simulink model "Simulink_Vortex"  (R2015b)
settings: Solver=ode3  StartTime=0.0  StopTime=20.603  FixedStep=0.016666  RelTol=1e-3
InitFcn:
  | state=0
values from neighbouring files (symbols this model uses):
  acc = 2    [sim_ExoTeR_VORTEX.m]
  mode = 0    [sim_ExoTeR_VORTEX.m]
libraries: simulink x6, Vortex x1
settings Model: Creator=pablorm  LastModifiedBy=gonzalopd96
settings RTWCC: PostCodeGenCommand=PrepareVortexForSimulinkCoder(buildInfo)

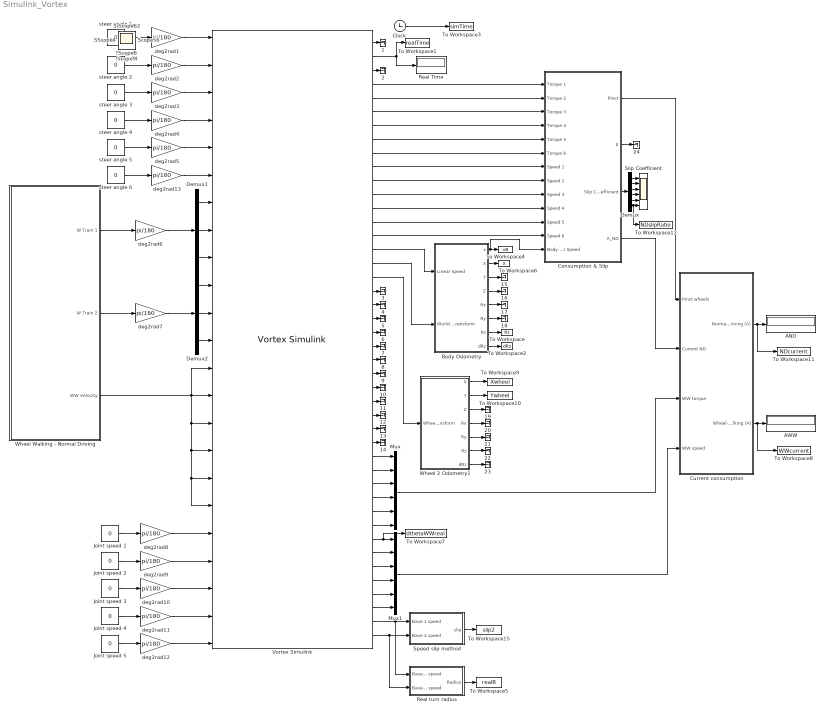
== system Simulink_Vortex ==
  {1..24} (24 alike) : Terminator
  AND : Display
  AWW : Display
  Body Odometry : Subsystem
  Clock : Clock
  Consumption & Slip : Subsystem
  Current consumption : Subsystem
  Demux : Demux  Outputs=6
  Demux1 : Demux  Outputs=3
  Demux2 : Demux  Outputs=3
  Joint speed {1..5} (5 alike) : Constant  Value=0
  Mux : Mux  Inputs=6
  Mux1 : Mux  Inputs=6
  Real Time : Display
  "Real turn radius " : Subsystem
  Slip Coefficient : Scope  NumInputPorts=6
  Speed slip method : Subsystem
  To Workspace : ToWorkspace  VariableName=Rz  SampleTime=-1
  To Workspace1 : ToWorkspace  VariableName=realTime  SampleTime=-1
  To Workspace10 : ToWorkspace  VariableName=Ywheel  SampleTime=-1
  To Workspace11 : ToWorkspace  VariableName=NDcurrent  SampleTime=-1
  To Workspace12 : ToWorkspace  VariableName=NDslipRatio  SampleTime=-1
  To Workspace15 : ToWorkspace  VariableName=slip2  SampleTime=-1
  To Workspace2 : ToWorkspace  VariableName=dRz  SampleTime=-1
  To Workspace3 : ToWorkspace  VariableName=simTime  SampleTime=-1
  To Workspace4 : ToWorkspace  VariableName=vB  SampleTime=-1
  To Workspace5 : ToWorkspace  VariableName=realR  SampleTime=-1
  To Workspace6 : ToWorkspace  VariableName=X  SampleTime=-1
  To Workspace7 : ToWorkspace  VariableName=dthetaWWreal  SampleTime=-1
      settings: Save2DSignal=2-D array (concatenate along first dimension)
  To Workspace8 : ToWorkspace  VariableName=WWcurrent  SampleTime=-1
  To Workspace9 : ToWorkspace  VariableName=Xwheel  SampleTime=-1
  Vortex Simulink : Vortex/Vortex Simulink  ip='127.0.0.1'  port='736'  path='C:\Users\gonzalopd96\Documents\VortexSimulink\Simulink\Simulink configurations\Rover_config.json'  display=image(imread('logo.jpg'), [0, 0, 48, 48]);fprintf('\n\n\nMy Model');port_label('input',1,'Steer1Angle');port_label('input',2,'Steer2Angle');port_label('input',3,'Steer3Angle');port_label('input',4,'Steer4Angle');port_label('input',5,'Steer5Angle');port_label('input',6,'Steer6Angle');port_label('input',7,'Speed1');port_label('input',8,'Speed2');port_label('input',9,'Speed3');port_label('input',10,'Speed4');port_label('input',11,'Speed5');port_label('input',12,'Speed6');port_label('input',13,'WJ1');port_label('input',14,'WJ2');port_label('input',15,'WJ3');port_label('input',16,'WJ4');port_label('input',17,'WJ5');port_label('input',18,'WJ6');port_label('input',19,'Joint speed 1');port_label('input',20,'Joint speed 2');port_label('input',21,'Joint speed 3');port_label('input',22,'Joint speed 4');port_label('input',23,'Joint speed 5');port_label('output',1,'Status');port_label('output',2,'Time');port_label('output',3,'FrameIndex');port_label('output',4,'Torque1');port_label('output',5,'Torque2');port_label('output',6,'Torque3');port_label('output',7,'Torque4');port_label('output',8,'Torque5');port_label('output',9,'Torque6');port_label('output',10,'Speed1');port_label('output',11,'Speed2');port_label('output',12,'Speed3');port_label('output',13,'Speed4');port_label('output',14,'Speed5');port_label('output',15,'Speed6');port_label('output',16,'Lineal Speed');port_label('output',17,'World Transform');port_label('output',18,'Wheel Transform');port_label('output',19,'Motor Transform');port_label('output',20,'PosJ1');port_label('output',21,'PosJ2');port_label('output',22,'PosJ3');port_label('output',23,'PosJ4');port_label('output',24,'PosJ5');port_label('output',25,'Steer1');port_label('output',26,'Steer2');port_label('output',27,'Steer3');port_label('output',28,'Steer4');port_label('output',29,'Steer5');port_label('output',30,'Steer6');port_label('output',31,'WW Torque 1');port_label('output',32,'WW Torque 2');port_label('output',33,'WW Torque 3');port_label('output',34,'WW Torque 4');port_label('output',35,'WW Torque 5');port_label('output',36,'WW Torque 6');port_label('output',37,'WW Speed 1');port_label('output',38,'WW Speed 2');port_label('output',39,'WW Speed 3');port_label('output',40,'WW Speed 4');port_label('output',41,'WW Speed 5');port_label('output',42,'WW Speed 6');port_label('output',43,'RS position');port_label('output',44,'LS position');  SynchronizationMechanism=Active wait at each step  WaitVortex=on
  Wheel 2 Odometry1 : Subsystem
  Wheel Walking - Normal Driving : Subsystem
  deg2rad{1..13} (13 alike) : Gain  Gain=pi/180
  steer angle {1..6} (6 alike) : Constant  Value=0
  Scope{,1..6,8..17} (17 alike) : Scope
  wires:
  deg2rad4/1 -> Vortex Simulink/4
  deg2rad3/1 -> Vortex Simulink/3
  deg2rad2/1 -> Vortex Simulink/2
  deg2rad5/1 -> Vortex Simulink/5
  deg2rad13/1 -> Vortex Simulink/6
  Joint speed 1/1 -> deg2rad8/1
  Joint speed 2/1 -> deg2rad9/1
  Joint speed 3/1 -> deg2rad10/1
  Joint speed 4/1 -> deg2rad11/1
  Joint speed 5/1 -> deg2rad12/1
  Vortex Simulink/4 -> Consumption & Slip/1(Torque 1)
  Vortex Simulink/6 -> Consumption & Slip/3(Torque 3)
  Vortex Simulink/7 -> Consumption & Slip/4(Torque 4)
  Vortex Simulink/8 -> Consumption & Slip/5(Torque 5)
  Vortex Simulink/9 -> Consumption & Slip/6(Torque 6)
  Vortex Simulink/10 -> Consumption & Slip/7(Speed 1)
  Vortex Simulink/11 -> Consumption & Slip/8(Speed 2)
  Vortex Simulink/12 -> Consumption & Slip/9(Speed 3)
  Vortex Simulink/13 -> Consumption & Slip/10(Speed 4)
  Vortex Simulink/14 -> Consumption & Slip/11(Speed 5)
  Vortex Simulink/15 -> Consumption & Slip/12(Speed 6)
  Body Odometry/1(v) -> Consumption & Slip/13(Body Linear Speed), To Workspace4/1
  Vortex Simulink/16 -> Body Odometry/1(Linear Speed)
  steer angle 6/1 -> deg2rad13/1
  steer angle 2/1 -> deg2rad2/1
  steer angle 3/1 -> deg2rad3/1
  steer angle 4/1 -> deg2rad4/1
  steer angle 5/1 -> deg2rad5/1
  Wheel Walking - Normal Driving/1(W Train 1) -> deg2rad6/1
  Wheel Walking - Normal Driving/2(W Train 2) -> deg2rad7/1
  Vortex Simulink/17 -> Body Odometry/2(World transform)
  Demux1/3 -> Vortex Simulink/9
  Demux1/2 -> Vortex Simulink/8
  deg2rad6/1 -> Demux1/1
  Demux2/2 -> Vortex Simulink/11
  Demux2/1 -> Vortex Simulink/10
  Demux2/3 -> Vortex Simulink/12
  deg2rad7/1 -> Demux2/1
  Consumption & Slip/3(Slip Coefficient) -> Demux/1
  Demux/1 -> Slip Coefficient/1
  Demux/2 -> Slip Coefficient/2
  Demux/3 -> Slip Coefficient/3
  Demux/4 -> Slip Coefficient/4
  Demux/5 -> Slip Coefficient/5
  Demux/6 -> To Workspace12/1, Slip Coefficient/6
  Vortex Simulink/2 -> To Workspace1/1, Real Time/1
  Demux1/1 -> Vortex Simulink/7
  Vortex Simulink/5 -> Consumption & Slip/2(Torque 2)
  Clock/1 -> To Workspace3/1
  Body Odometry/2(X) -> To Workspace6/1
  Body Odometry/7(Rz) -> To Workspace/1
  Body Odometry/8(dRz) -> To Workspace2/1
  Wheel 2 Odometry1/2(Y) -> To Workspace10/1
  Wheel 2 Odometry1/1(X) -> To Workspace9/1
  Speed slip method/1(slip) -> To Workspace15/1
  Consumption & Slip/1(PInst) -> Current consumption/1(Pinst wheels)
  Consumption & Slip/4(A_ND) -> Current consumption/2(Current ND)
  Mux/1 -> Current consumption/3(WW torque)
  Mux1/1 -> Current consumption/4(WW speed)
  Current consumption/1(Normal driving (A)) -> To Workspace11/1, AND/1
  Current consumption/2(Wheel-walking (A)) -> To Workspace8/1, AWW/1
  deg2rad1/1 -> Vortex Simulink/1
  steer angle 1/1 -> deg2rad1/1
  Body Odometry/4(Z) -> 16/1
  Body Odometry/6(Ry) -> 18/1
  Body Odometry/5(Rx) -> 17/1
  Body Odometry/3(Y) -> 15/1
  Consumption & Slip/2(P) -> 24/1
  Vortex Simulink/1 -> 1/1
  Vortex Simulink/3 -> 2/1
  Wheel 2 Odometry1/3(Z) -> 19/1
  Wheel 2 Odometry1/4(Rx) -> 20/1
  Wheel 2 Odometry1/5(Ry) -> 21/1
  Wheel 2 Odometry1/6(Rz) -> 22/1
  Wheel 2 Odometry1/7(dRz) -> 23/1
  "Real turn radius "/1(Radius) -> To Workspace5/1
  Wheel Walking - Normal Driving/3(WW Velocity) -> Vortex Simulink/14, Vortex Simulink/13, Vortex Simulink/15, Vortex Simulink/16, Vortex Simulink/18, Vortex Simulink/17
  deg2rad8/1 -> Vortex Simulink/19
  deg2rad9/1 -> Vortex Simulink/20
  deg2rad10/1 -> Vortex Simulink/21
  deg2rad11/1 -> Vortex Simulink/22
  deg2rad12/1 -> Vortex Simulink/23
  Vortex Simulink/43 -> "Real turn radius "/1(Base 1 speed), Speed slip method/1(Base 1 speed)
  Vortex Simulink/44 -> "Real turn radius "/2(Base 2 speed), Speed slip method/2(Base 2 speed)
  Vortex Simulink/18 -> Wheel 2 Odometry1/1(Wheel transform)
  Vortex Simulink/19 -> 3/1
  Vortex Simulink/20 -> 4/1
  Vortex Simulink/21 -> 5/1
  Vortex Simulink/22 -> 6/1
  Vortex Simulink/23 -> 7/1
  Vortex Simulink/24 -> 8/1
  Vortex Simulink/25 -> 9/1
  Vortex Simulink/26 -> 10/1
  Vortex Simulink/27 -> 11/1
  Vortex Simulink/28 -> 12/1
  Vortex Simulink/29 -> 13/1
  Vortex Simulink/30 -> 14/1
  Vortex Simulink/36 -> Mux/6
  Vortex Simulink/35 -> Mux/5
  Vortex Simulink/34 -> Mux/4
  Vortex Simulink/33 -> Mux/3
  Vortex Simulink/32 -> Mux/2
  Vortex Simulink/31 -> Mux/1
  Vortex Simulink/38 -> Mux1/2
  Vortex Simulink/39 -> Mux1/3
  Vortex Simulink/40 -> Mux1/4
  Vortex Simulink/41 -> Mux1/5
  Vortex Simulink/42 -> Mux1/6
  Vortex Simulink/37 -> To Workspace7/1, Mux1/1

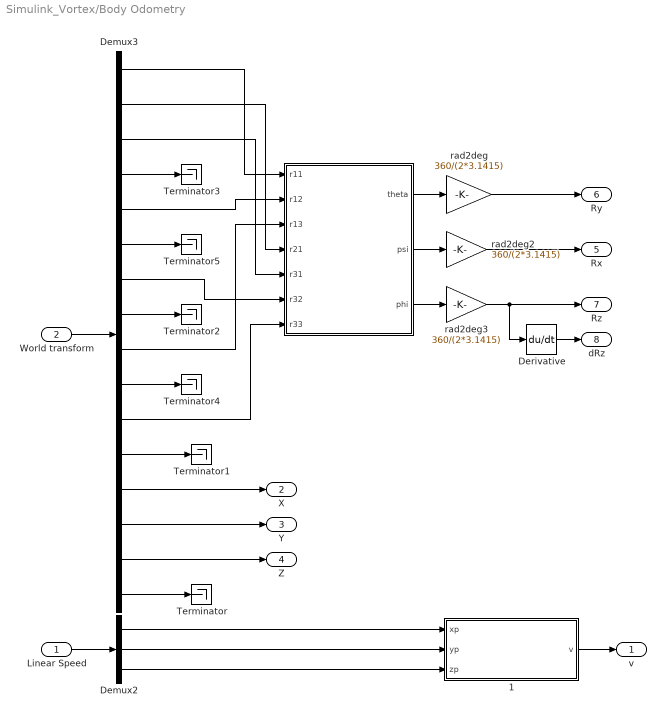
== system Simulink_Vortex/Body Odometry ==
  Linear Speed : Inport
  World transform : Inport  Port=2
  " " : MATLAB Function  TreatAsAtomicUnit=on
  1 : MATLAB Function  TreatAsAtomicUnit=on
  Demux2 : Demux  Outputs=3
  Demux3 : Demux  Outputs=16
  Derivative : Derivative
  Terminator{,1..5} (6 alike) : Terminator
  rad2deg : Gain  Gain=360/(2*3.1415)
  rad2deg2 : Gain  Gain=360/(2*3.1415)
  rad2deg3 : Gain  Gain=360/(2*3.1415)
  v : Outport
  X : Outport  Port=2
  Y : Outport  Port=3
  Z : Outport  Port=4
  Rx : Outport  Port=5
  Ry : Outport  Port=6
  Rz : Outport  Port=7
  dRz : Outport  Port=8
  wires:
  World transform/1 -> Demux3/1
  Demux3/13 -> X/1
  Demux3/14 -> Y/1
  Demux3/15 -> Z/1
  Demux3/7 -> " "/6(r32)
  Demux3/6 -> Terminator5/1
  " "/2(psi) -> rad2deg2/1
  " "/1(theta) -> rad2deg/1
  Demux3/4 -> Terminator3/1
  " "/3(phi) -> rad2deg3/1
  Demux3/12 -> Terminator1/1
  Demux3/16 -> Terminator/1
  rad2deg3/1 -> Derivative/1, Rz/1
  rad2deg2/1 -> Rx/1
  rad2deg/1 -> Ry/1
  Linear Speed/1 -> Demux2/1
  Demux2/1 -> 1/1(xp)
  1/1(v) -> v/1
  Demux2/2 -> 1/2(yp)
  Demux2/3 -> 1/3(zp)
  Derivative/1 -> dRz/1
  Demux3/1 -> " "/1(r11)
  Demux3/2 -> " "/4(r21)
  Demux3/3 -> " "/5(r31)
  Demux3/5 -> " "/2(r12)
  Demux3/8 -> Terminator2/1
  Demux3/9 -> " "/3(r13)
  Demux3/10 -> Terminator4/1
  Demux3/11 -> " "/7(r33)

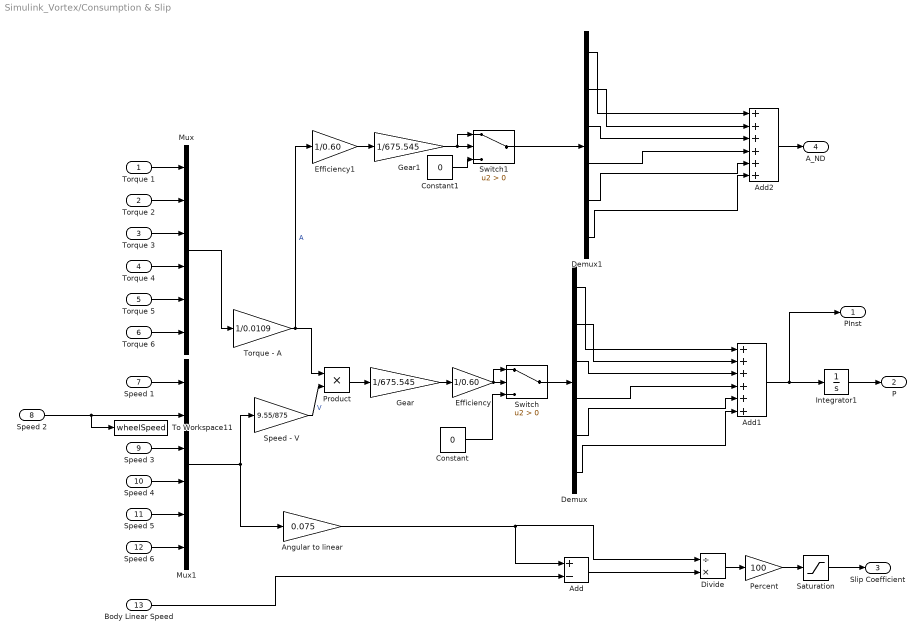
== system Simulink_Vortex/Consumption & Slip ==
  Torque 1 : Inport
  Torque 2 : Inport  Port=2
  Torque 3 : Inport  Port=3
  Torque 4 : Inport  Port=4
  Torque 5 : Inport  Port=5
  Torque 6 : Inport  Port=6
  Speed 1 : Inport  Port=7
  Speed 2 : Inport  Port=8
  Speed 3 : Inport  Port=9
  Speed 4 : Inport  Port=10
  Speed 5 : Inport  Port=11
  Speed 6 : Inport  Port=12
  Body Linear Speed : Inport  Port=13
  Add : Sum  Inputs=+-
  Add1 : Sum  Inputs=++++++
  Add2 : Sum  Inputs=++++++
  Angular to linear : Gain  Gain=0.075
  Constant : Constant  Value=0
  Constant1 : Constant  Value=0
  Demux : Demux  Outputs=6
  Demux1 : Demux  Outputs=6
  Divide : Product  Inputs=/*
  Efficiency : Gain  Gain=1/0.60
  Efficiency1 : Gain  Gain=1/0.60
  Gear : Gain  Gain=1/675.545
  Gear1 : Gain  Gain=1/675.545
  Integrator1 : Integrator
  Mux : Mux  Inputs=6
  Mux1 : Mux  Inputs=6
  Percent : Gain  Gain=100
  Product : Product
  Saturation : Saturate  UpperLimit=100  LowerLimit=0
  Speed - V : Gain  Gain=9.55/875
  Switch : Switch  Criteria=u2 > Threshold
  Switch1 : Switch  Criteria=u2 > Threshold
  To Workspace11 : ToWorkspace  VariableName=wheelSpeed  SampleTime=-1
  Torque - A : Gain  Gain=1/0.0109
  PInst : Outport
  P : Outport  Port=2
  Slip Coefficient : Outport  Port=3
  A_ND : Outport  Port=4
  wires:
  Torque 4/1 -> Mux/4
  Speed 4/1 -> Mux1/4
  Torque 3/1 -> Mux/3
  Torque 2/1 -> Mux/2
  Speed 6/1 -> Mux1/6
  Efficiency/1 -> Switch/1, Switch/2
  Torque 5/1 -> Mux/5
  Integrator1/1 -> P/1
  Torque 6/1 -> Mux/6
  Torque 1/1 -> Mux/1
  Demux/2 -> Add1/2
  Add1/1 -> PInst/1, Integrator1/1
  Torque - A/1 -> Product/1, Efficiency1/1  "A"
  Speed 1/1 -> Mux1/1
  Demux/4 -> Add1/4
  Speed 5/1 -> Mux1/5
  Demux/6 -> Add1/6
  Demux/3 -> Add1/3
  Speed - V/1 -> Product/2  "V"
  Speed 3/1 -> Mux1/3
  Demux/5 -> Add1/5
  Demux/1 -> Add1/1
  Mux1/1 -> Angular to linear/1, Speed - V/1
  Body Linear Speed/1 -> Add/2
  Divide/1 -> Percent/1
  Percent/1 -> Saturation/1
  Saturation/1 -> Slip Coefficient/1
  Add/1 -> Divide/2
  Angular to linear/1 -> Add/1, Divide/1
  Mux/1 -> Torque - A/1
  Switch/1 -> Demux/1
  Constant/1 -> Switch/3
  Product/1 -> Gear/1
  Gear/1 -> Efficiency/1
  Demux1/2 -> Add2/2
  Demux1/4 -> Add2/4
  Demux1/6 -> Add2/6
  Demux1/3 -> Add2/3
  Demux1/5 -> Add2/5
  Demux1/1 -> Add2/1
  Add2/1 -> A_ND/1
  Switch1/1 -> Demux1/1
  Constant1/1 -> Switch1/3
  Gear1/1 -> Switch1/1, Switch1/2
  Efficiency1/1 -> Gear1/1
  Speed 2/1 -> To Workspace11/1, Mux1/2

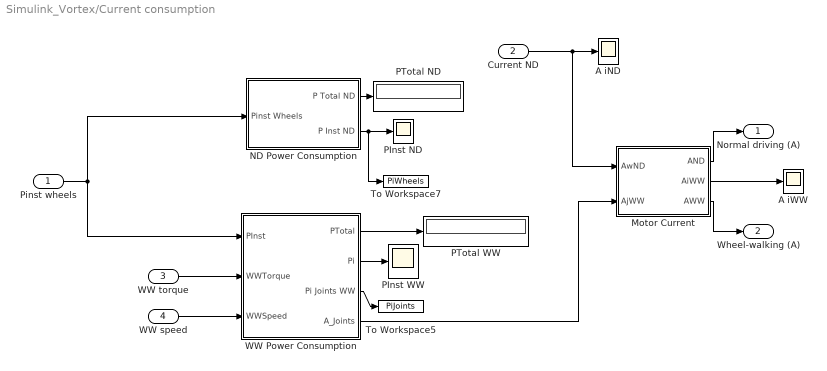
== system Simulink_Vortex/Current consumption ==
  Pinst wheels : Inport
  Current ND : Inport  Port=2
  WW torque : Inport  Port=3
  WW speed : Inport  Port=4
  A iND : Scope
  A iWW : Scope
  Motor Current : Subsystem
  ND Power Consumption : Subsystem
  PInst ND : Scope
  PInst WW : Scope
  PTotal ND : Display
  PTotal WW : Display
  To Workspace5 : ToWorkspace  VariableName=PiJoints  SampleTime=-1
  To Workspace7 : ToWorkspace  VariableName=PiWheels  SampleTime=-1
  WW Power Consumption : Subsystem
  Normal driving (A) : Outport
  Wheel-walking (A) : Outport  Port=2
  wires:
  Pinst wheels/1 -> ND Power Consumption/1(Pinst Wheels), WW Power Consumption/1(PInst)
  WW torque/1 -> WW Power Consumption/2(WWTorque)
  WW Power Consumption/2(Pi) -> PInst WW/1
  WW Power Consumption/1(PTotal) -> PTotal WW/1
  ND Power Consumption/1(P Total ND) -> PTotal ND/1
  ND Power Consumption/2(P Inst ND) -> To Workspace7/1, PInst ND/1
  WW Power Consumption/3(Pi Joints WW) -> To Workspace5/1
  WW speed/1 -> WW Power Consumption/3(WWSpeed)
  Current ND/1 -> Motor Current/1(AwND), A iND/1
  WW Power Consumption/4(A_Joints) -> Motor Current/2(AjWW)
  Motor Current/1(AND) -> Normal driving (A)/1
  Motor Current/3(AWW) -> Wheel-walking (A)/1
  Motor Current/2(AiWW) -> A iWW/1

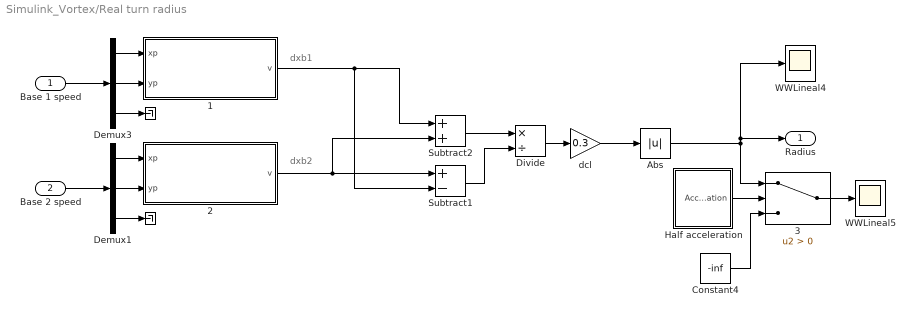
== system Simulink_Vortex/Real turn radius  ==
  note: dxb2
  note: dxb1
  Base 1 speed : Inport
  Base 2 speed : Inport  Port=2
  " " : Terminator
  " " : Terminator
  "     3" : Switch  Criteria=u2 > Threshold
  1 : MATLAB Function  TreatAsAtomicUnit=on
  2 : MATLAB Function  TreatAsAtomicUnit=on
  Abs : Abs
  Constant4 : Constant  Value=-inf
  Demux1 : Demux  Outputs=3
  Demux3 : Demux  Outputs=3
  Divide : Product  Inputs=*/
  Half acceleration : Subsystem
  Subtract1 : Sum  Inputs=+-
  Subtract2 : Sum
  WWLineal4 : Scope
  WWLineal5 : Scope
  dcl : Gain  Gain=0.3
  Radius : Outport
  wires:
  Half acceleration/1(Acceleration) -> "     3"/2
  Divide/1 -> dcl/1
  Constant4/1 -> "     3"/3
  "     3"/1 -> WWLineal5/1
  1/1(v) -> Subtract2/1, Subtract1/2
  dcl/1 -> Abs/1
  Abs/1 -> WWLineal4/1, Radius/1, "     3"/1
  Subtract1/1 -> Divide/2
  Subtract2/1 -> Divide/1
  Base 1 speed/1 -> Demux3/1
  Demux3/2 -> 1/2(yp)
  Demux3/1 -> 1/1(xp)
  Demux3/3 -> " "/1
  Base 2 speed/1 -> Demux1/1
  Demux1/2 -> 2/2(yp)
  Demux1/1 -> 2/1(xp)
  Demux1/3 -> " "/1
  2/1(v) -> Subtract1/1, Subtract2/2

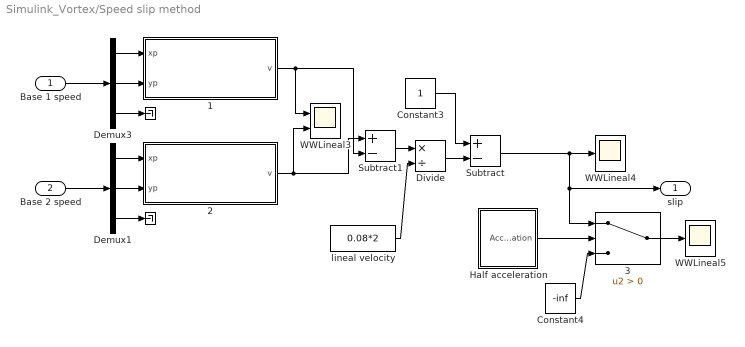
== system Simulink_Vortex/Speed slip method ==
  Base 1 speed : Inport
  Base 2 speed : Inport  Port=2
  " " : Terminator
  " " : Terminator
  "     3" : Switch  Criteria=u2 > Threshold
  1 : MATLAB Function  TreatAsAtomicUnit=on
  2 : MATLAB Function  TreatAsAtomicUnit=on
  Constant3 : Constant
  Constant4 : Constant  Value=-inf
  Demux1 : Demux  Outputs=3
  Demux3 : Demux  Outputs=3
  Divide : Product  Inputs=*/
  Half acceleration : Subsystem
  Subtract : Sum  Inputs=+-
  Subtract1 : Sum  Inputs=+-
  WWLineal3 : Scope  NumInputPorts=2
  WWLineal4 : Scope
  WWLineal5 : Scope
  lineal velocity : Constant  Value=0.08*2
  slip : Outport
  wires:
  Half acceleration/1(Acceleration) -> "     3"/2
  Constant3/1 -> Subtract/1
  Subtract1/1 -> Divide/1
  Divide/1 -> Subtract/2
  lineal velocity/1 -> Divide/2
  Constant4/1 -> "     3"/3
  "     3"/1 -> WWLineal5/1
  2/1(v) -> Subtract1/1, WWLineal3/2
  Subtract/1 -> WWLineal4/1, slip/1, "     3"/1
  1/1(v) -> Subtract1/2, WWLineal3/1
  Base 1 speed/1 -> Demux3/1
  Demux3/2 -> 1/2(yp)
  Demux3/1 -> 1/1(xp)
  Demux3/3 -> " "/1
  Base 2 speed/1 -> Demux1/1
  Demux1/2 -> 2/2(yp)
  Demux1/1 -> 2/1(xp)
  Demux1/3 -> " "/1

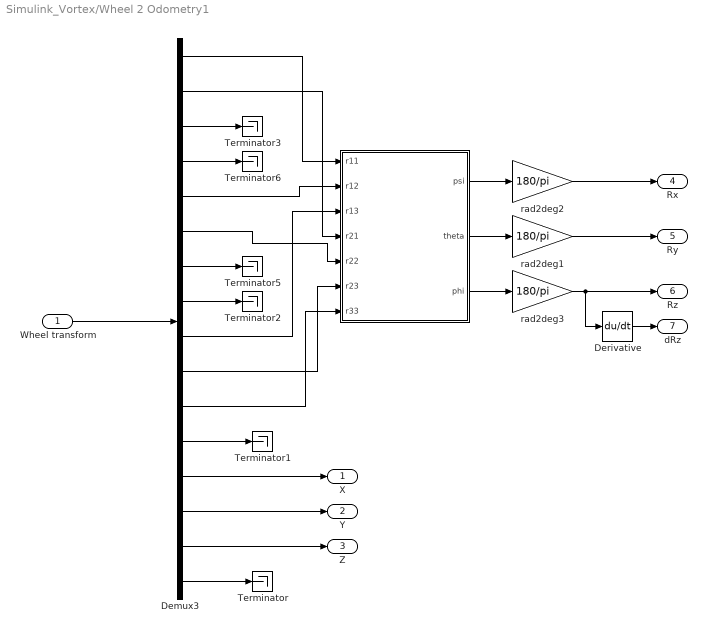
== system Simulink_Vortex/Wheel 2 Odometry1 ==
  Wheel transform : Inport
  " " : MATLAB Function  TreatAsAtomicUnit=on
  Demux3 : Demux  Outputs=16
  Derivative : Derivative
  Terminator{,1..3,5..6} (6 alike) : Terminator
  rad2deg1 : Gain  Gain=180/pi
  rad2deg2 : Gain  Gain=180/pi
  rad2deg3 : Gain  Gain=180/pi
  X : Outport
  Y : Outport  Port=2
  Z : Outport  Port=3
  Rx : Outport  Port=4
  Ry : Outport  Port=5
  Rz : Outport  Port=6
  dRz : Outport  Port=7
  wires:
  Derivative/1 -> dRz/1
  rad2deg1/1 -> Ry/1
  rad2deg2/1 -> Rx/1
  rad2deg3/1 -> Rz/1, Derivative/1
  Demux3/16 -> Terminator/1
  " "/3(phi) -> rad2deg3/1
  " "/2(theta) -> rad2deg1/1
  " "/1(psi) -> rad2deg2/1
  Demux3/15 -> Z/1
  Demux3/14 -> Y/1
  Demux3/13 -> X/1
  Wheel transform/1 -> Demux3/1
  Demux3/12 -> Terminator1/1
  Demux3/8 -> Terminator2/1
  Demux3/1 -> " "/1(r11)
  Demux3/2 -> " "/4(r21)
  Demux3/3 -> Terminator3/1
  Demux3/4 -> Terminator6/1
  Demux3/5 -> " "/2(r12)
  Demux3/6 -> " "/5(r22)
  Demux3/7 -> Terminator5/1
  Demux3/9 -> " "/3(r13)
  Demux3/10 -> " "/6(r23)
  Demux3/11 -> " "/7(r33)

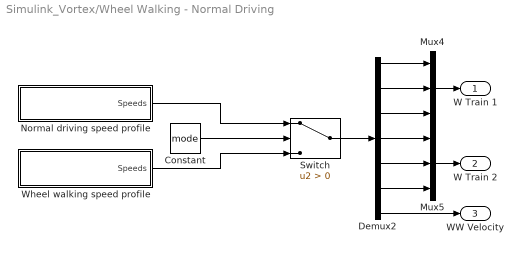
== system Simulink_Vortex/Wheel Walking - Normal Driving ==
  Constant : Constant  Value=mode
  Demux2 : Demux  Outputs=7
  Mux4 : Mux  Inputs=3
  Mux5 : Mux  Inputs=3
  Normal driving speed profile : Subsystem
  Switch : Switch  Criteria=u2 > Threshold
  Wheel walking speed profile : Subsystem
  W Train 1 : Outport
  W Train 2 : Outport  Port=2
  WW Velocity : Outport  Port=3
  wires:
  Demux2/1 -> Mux4/1
  Demux2/2 -> Mux4/2
  Demux2/3 -> Mux4/3
  Demux2/6 -> Mux5/3
  Demux2/5 -> Mux5/2
  Demux2/4 -> Mux5/1
  Mux4/1 -> W Train 1/1
  Mux5/1 -> W Train 2/1
  Demux2/7 -> WW Velocity/1
  Switch/1 -> Demux2/1
  Normal driving speed profile/1(Speeds) -> Switch/1
  Wheel walking speed profile/1(Speeds) -> Switch/3
  Constant/1 -> Switch/2

== system Simulink_Vortex/Current consumption/Motor Current ==
  AwND : Inport
  AjWW : Inport  Port=2
  Add3 : Sum
  Integrator : Integrator
  Integrator1 : Integrator
  AND : Outport
  AiWW : Outport  Port=2
  AWW : Outport  Port=3
  wires:
  Integrator1/1 -> AWW/1
  AjWW/1 -> Add3/2
  Integrator/1 -> AND/1
  Add3/1 -> AiWW/1, Integrator1/1
  AwND/1 -> Integrator/1, Add3/1

== system Simulink_Vortex/Current consumption/ND Power Consumption ==
  Pinst Wheels : Inport
  Gain : Gain
  Integrator : Integrator
  P Total ND : Outport
  P Inst ND : Outport  Port=2
  wires:
  Pinst Wheels/1 -> P Inst ND/1, Gain/1
  Gain/1 -> Integrator/1
  Integrator/1 -> P Total ND/1

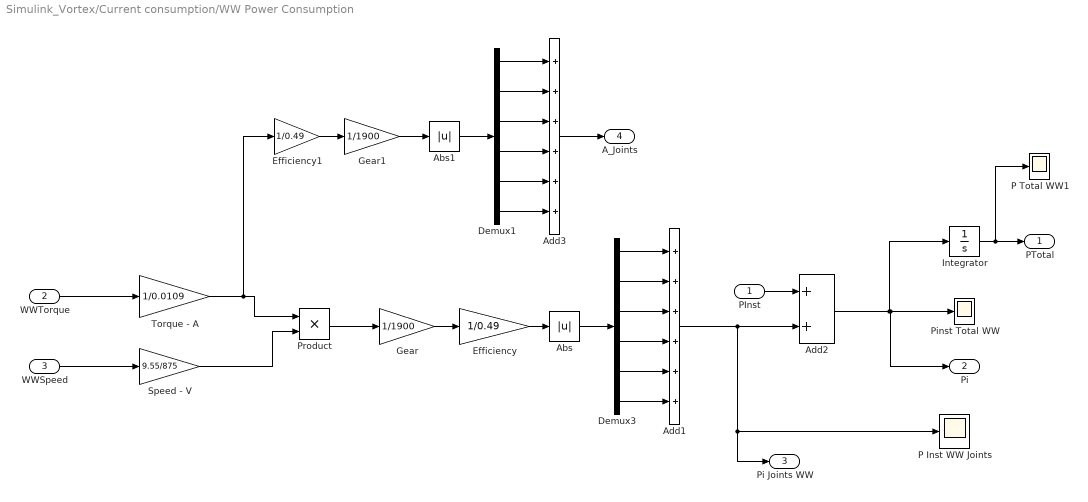
== system Simulink_Vortex/Current consumption/WW Power Consumption ==
  PInst : Inport
  WWTorque : Inport  Port=2
  WWSpeed : Inport  Port=3
  Abs : Abs
  Abs1 : Abs
  Add1 : Sum  Inputs=++++++
  Add2 : Sum
  Add3 : Sum  Inputs=++++++
  Demux1 : Demux  Outputs=6
  Demux3 : Demux  Outputs=6
  Efficiency : Gain  Gain=1/0.49
  Efficiency1 : Gain  Gain=1/0.49
  Gear : Gain  Gain=1/1900
  Gear1 : Gain  Gain=1/1900
  Integrator : Integrator
  P Inst WW Joints : Scope
  P Total WW1 : Scope
  Pinst Total WW : Scope
  Product : Product
  Speed - V : Gain  Gain=9.55/875
  Torque - A : Gain  Gain=1/0.0109
  PTotal : Outport
  Pi : Outport  Port=2
  Pi Joints WW : Outport  Port=3
  A_Joints : Outport  Port=4
  wires:
  PInst/1 -> Add2/1
  WWTorque/1 -> Torque - A/1
  Efficiency/1 -> Abs/1
  Demux3/1 -> Add1/1
  Demux3/2 -> Add1/2
  Demux3/3 -> Add1/3
  Demux3/4 -> Add1/4
  Demux3/5 -> Add1/5
  Demux3/6 -> Add1/6
  Abs/1 -> Demux3/1
  Add1/1 -> Pi Joints WW/1, P Inst WW Joints/1, Add2/2
  Add2/1 -> Pinst Total WW/1, Pi/1, Integrator/1
  Integrator/1 -> P Total WW1/1, PTotal/1
  Gear/1 -> Efficiency/1
  WWSpeed/1 -> Speed - V/1
  Speed - V/1 -> Product/2
  Product/1 -> Gear/1
  Demux1/1 -> Add3/1
  Demux1/2 -> Add3/2
  Demux1/3 -> Add3/3
  Demux1/4 -> Add3/4
  Demux1/5 -> Add3/5
  Demux1/6 -> Add3/6
  Torque - A/1 -> Efficiency1/1, Product/1
  Add3/1 -> A_Joints/1
  Abs1/1 -> Demux1/1
  Gear1/1 -> Abs1/1
  Efficiency1/1 -> Gear1/1

== system Simulink_Vortex/Real turn radius /Half acceleration ==
  Constant : Constant
  Constant2 : Constant  Value=0.4
  Divide : Product  Inputs=*/
  Repeating Sequence : simulink/Sources/Repeating Sequence  rep_seq_t=[0.665 14.63 14.63+0.000001 15.96 15.96+0.000001]  rep_seq_y=[1 1 2 2 1]
  Subtract : Sum  Inputs=+-
  Acceleration : Outport
  wires:
  Constant/1 -> Subtract/2
  Subtract/1 -> Divide/1
  Repeating Sequence/1 -> Subtract/1
  Constant2/1 -> Divide/2
  Divide/1 -> Acceleration/1

== system Simulink_Vortex/Speed slip method/Half acceleration ==
  Constant : Constant
  Constant2 : Constant  Value=0.4
  Divide : Product  Inputs=*/
  Repeating Sequence : simulink/Sources/Repeating Sequence  rep_seq_t=[0.665 14.63 14.63+0.000001 15.96 15.96+0.000001]  rep_seq_y=[1 1 2 2 1]
  Subtract : Sum  Inputs=+-
  Acceleration : Outport
  wires:
  Constant/1 -> Subtract/2
  Subtract/1 -> Divide/1
  Repeating Sequence/1 -> Subtract/1
  Constant2/1 -> Divide/2
  Divide/1 -> Acceleration/1

== system Simulink_Vortex/Wheel Walking - Normal Driving/Normal driving speed profile ==
  "       1/r" : Gain  Gain=1/0.075
  Mux : Mux  Inputs=3
  Mux6 : Mux  Inputs=3
  Mux7 : Mux  Inputs=3
  WWalking : Constant  Value=0
  lineal velocity : Constant  Value=0.08
  rad2grad : Gain  Gain=180/pi
  Speeds : Outport
  wires:
  Mux/1 -> Speeds/1
  WWalking/1 -> Mux/3
  "       1/r"/1 -> rad2grad/1
  Mux6/1 -> Mux/1
  Mux7/1 -> Mux/2
  lineal velocity/1 -> "       1/r"/1
  rad2grad/1 -> Mux6/2, Mux7/3, Mux7/2, Mux7/1, Mux6/3, Mux6/1

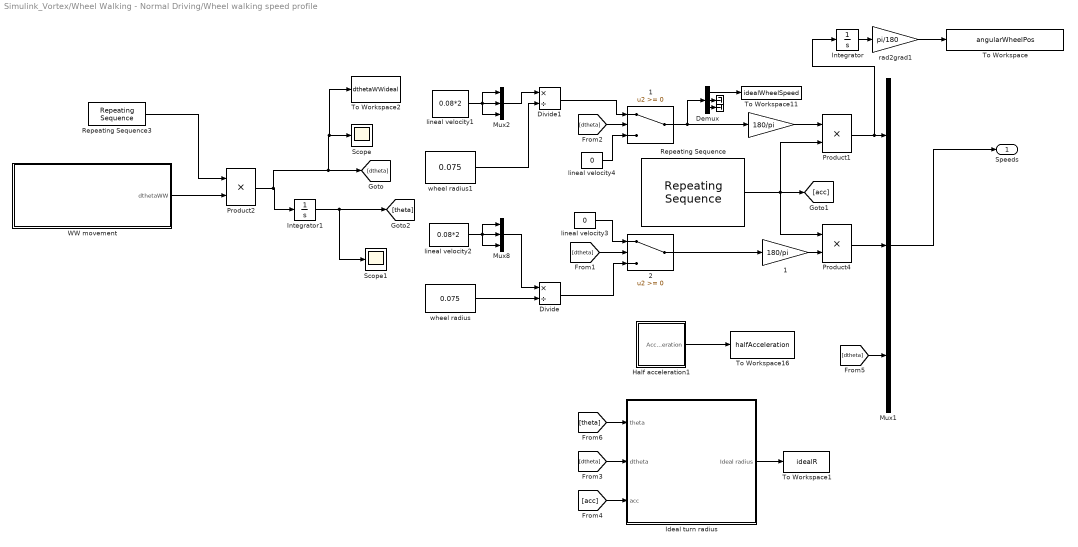
== system Simulink_Vortex/Wheel Walking - Normal Driving/Wheel walking speed profile ==
  " " : Terminator
  " " : Terminator
  " " : Gain  Gain=180/pi
  "       1" : Gain  Gain=180/pi
  "     1" : Switch
  "     2" : Switch
  Demux : Demux  Outputs=3
  Divide : Product  Inputs=*/
  Divide1 : Product  Inputs=*/
  Half acceleration1 : Subsystem
  Ideal turn radius : Subsystem
  Integrator : Integrator
  Integrator1 : Integrator
  Mux1 : Mux  Inputs=3
  Mux2 : Mux  Inputs=3
  Mux8 : Mux  Inputs=3
  Product1 : Product
  Product2 : Product
  Product4 : Product
  Repeating Sequence : simulink/Sources/Repeating Sequence  rep_seq_t=[0.665 14.63 14.63+0.000001 17.29 17.29+0.000001]  rep_seq_y=[1 1 acc acc 1]
  Repeating Sequence3 : simulink/Sources/Repeating Sequence  rep_seq_t=[0.668 1.317 1.317+eps 1.317+2*eps 2.001]  rep_seq_y=[1 1 -1 1 1]
  Scope : Scope
  Scope1 : Scope
  To Workspace : ToWorkspace  VariableName=angularWheelPos  SampleTime=-1
      settings: Save2DSignal=2-D array (concatenate along first dimension)
  To Workspace1 : ToWorkspace  VariableName=idealR  SampleTime=-1
      settings: Save2DSignal=2-D array (concatenate along first dimension)
  To Workspace11 : ToWorkspace  VariableName=idealWheelSpeed  SampleTime=-1
      settings: Save2DSignal=2-D array (concatenate along first dimension)
  To Workspace16 : ToWorkspace  VariableName=halfAcceleration  SampleTime=-1
  To Workspace2 : ToWorkspace  VariableName=dthetaWWideal  SampleTime=-1
      settings: Save2DSignal=2-D array (concatenate along first dimension)
  WW movement : Subsystem
  lineal velocity1 : Constant  Value=0.08*2
  lineal velocity2 : Constant  Value=0.08*2
  lineal velocity3 : Constant  Value=0
  lineal velocity4 : Constant  Value=0
  rad2grad1 : Gain  Gain=pi/180
  wheel radius : Constant  Value=0.075
  wheel radius1 : Constant  Value=0.075
  Speeds : Outport
  wires:
  Mux1/1 -> Speeds/1
  wheel radius/1 -> Divide/2
  Mux8/1 -> Divide/1
  lineal velocity2/1 -> Mux8/1, Mux8/3, Mux8/2
  Product4/1 -> Mux1/2
  Product1/1 -> Integrator/1, Mux1/1
  " "/1 -> Product1/1
  Integrator/1 -> rad2grad1/1
  rad2grad1/1 -> To Workspace/1
  Repeating Sequence/1 -> [acc], Product4/1, Product1/2
  "       1"/1 -> Product4/2
  [dtheta] -> "     2"/2
  "     2"/1 -> "       1"/1
  wheel radius1/1 -> Divide1/2
  Mux2/1 -> Divide1/1
  lineal velocity1/1 -> Mux2/1, Mux2/3, Mux2/2
  [dtheta] -> "     1"/2
  "     1"/1 -> Demux/1, " "/1
  lineal velocity4/1 -> "     1"/3
  lineal velocity3/1 -> "     2"/1
  Divide1/1 -> "     1"/1
  Divide/1 -> "     2"/3
  Half acceleration1/1(Acceleration) -> To Workspace16/1
  [dtheta] -> Mux1/3
  [theta] -> Ideal turn radius/1(theta)
  [dtheta] -> Ideal turn radius/2(dtheta)
  [acc] -> Ideal turn radius/3(acc)
  Ideal turn radius/1(Ideal radius) -> To Workspace1/1
  Demux/1 -> To Workspace11/1
  Demux/2 -> " "/1
  Demux/3 -> " "/1
  Repeating Sequence3/1 -> Product2/1
  Integrator1/1 -> Scope1/1, [theta]
  WW movement/1(dthetaWW) -> Product2/2
  Product2/1 -> To Workspace2/1, Scope/1, [dtheta], Integrator1/1

== system Simulink_Vortex/Wheel Walking - Normal Driving/Wheel walking speed profile/Half acceleration1 ==
  Constant : Constant
  Constant2 : Constant  Value=0.4
  Divide : Product  Inputs=*/
  Repeating Sequence : simulink/Sources/Repeating Sequence  rep_seq_t=[0.665 14.63 14.63+0.000001 15.96 15.96+0.000001]  rep_seq_y=[1 1 2 2 1]
  Subtract : Sum  Inputs=+-
  Acceleration : Outport
  wires:
  Constant/1 -> Subtract/2
  Subtract/1 -> Divide/1
  Repeating Sequence/1 -> Subtract/1
  Constant2/1 -> Divide/2
  Divide/1 -> Acceleration/1

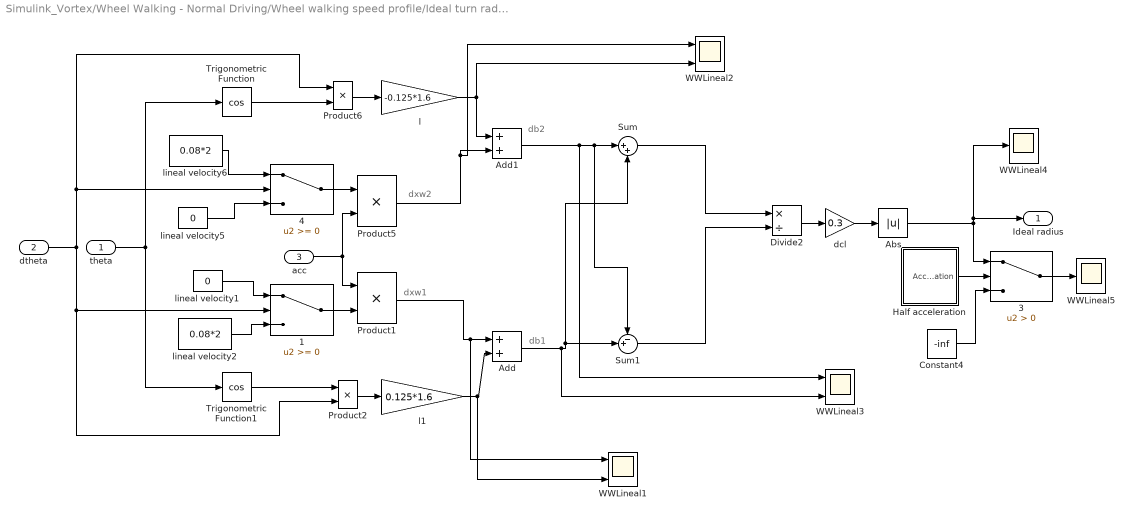
== system Simulink_Vortex/Wheel Walking - Normal Driving/Wheel walking speed profile/Ideal turn radius ==
  note: db2
  note: db1
  note: dxw1
  note: dxw2
  theta : Inport
  dtheta : Inport  Port=2
  acc : Inport  Port=3
  "     1" : Switch
  "     3" : Switch  Criteria=u2 > Threshold
  "     4" : Switch
  Abs : Abs
  Add : Sum
  Add1 : Sum
  Constant4 : Constant  Value=-inf
  Divide2 : Product  Inputs=*/
  Half acceleration : Subsystem
  Product{1..2,5..6} (4 alike) : Product
  Sum : Sum  Inputs=|++
  Sum1 : Sum  Inputs=-+|
  Trigonometric Function : Trigonometry  Operator=cos
  Trigonometric Function1 : Trigonometry  Operator=cos
  WWLineal1 : Scope  NumInputPorts=2
  WWLineal2 : Scope  NumInputPorts=2
  WWLineal3 : Scope  NumInputPorts=2
  WWLineal4 : Scope
  WWLineal5 : Scope
  dcl : Gain  Gain=0.3
  l : Gain  Gain=-0.125*1.6
  l1 : Gain  Gain=0.125*1.6
  lineal velocity1 : Constant  Value=0
  lineal velocity2 : Constant  Value=0.08*2
  lineal velocity5 : Constant  Value=0
  lineal velocity6 : Constant  Value=0.08*2
  Ideal radius : Outport
  wires:
  Product5/1 -> WWLineal2/1, Add1/2
  Trigonometric Function/1 -> Product6/2
  theta/1 -> Trigonometric Function/1, Trigonometric Function1/1
  "     4"/1 -> Product5/1
  acc/1 -> Product5/2, Product1/1
  Constant4/1 -> "     3"/3
  Half acceleration/1(Acceleration) -> "     3"/2
  Divide2/1 -> dcl/1
  "     3"/1 -> WWLineal5/1
  lineal velocity5/1 -> "     4"/3
  lineal velocity6/1 -> "     4"/1
  dtheta/1 -> "     4"/2, Product6/1, Product2/2, "     1"/2
  lineal velocity1/1 -> "     1"/1
  lineal velocity2/1 -> "     1"/3
  "     1"/1 -> Product1/2
  Product1/1 -> WWLineal1/1, Add/1
  dcl/1 -> Abs/1
  Product6/1 -> l/1
  Product2/1 -> l1/1
  Trigonometric Function1/1 -> Product2/1
  l1/1 -> WWLineal1/2, Add/2
  l/1 -> Add1/1, WWLineal2/2
  Sum/1 -> Divide2/1
  Sum1/1 -> Divide2/2
  Add1/1 -> WWLineal3/1, Sum1/1, Sum/1
  Add/1 -> WWLineal3/2, Sum/2, Sum1/2
  Abs/1 -> WWLineal4/1, Ideal radius/1, "     3"/1

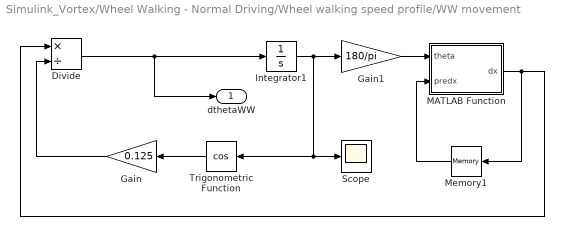
== system Simulink_Vortex/Wheel Walking - Normal Driving/Wheel walking speed profile/WW movement ==
  Divide : Product  Inputs=*/
  Gain : Gain  Gain=0.125
  Gain1 : Gain  Gain=180/pi
  Integrator1 : Integrator
  MATLAB Function : MATLAB Function  TreatAsAtomicUnit=on
  Memory1 : Memory  X0=-0.05
  Scope : Scope
  Trigonometric Function : Trigonometry  Operator=cos
  dthetaWW : Outport
  wires:
  MATLAB Function/1(dx) -> Memory1/1, Divide/1
  Gain1/1 -> MATLAB Function/1(theta)
  Integrator1/1 -> Trigonometric Function/1, Scope/1, Gain1/1
  Memory1/1 -> MATLAB Function/2(predx)
  Trigonometric Function/1 -> Gain/1
  Gain/1 -> Divide/2
  Divide/1 -> dthetaWW/1, Integrator1/1

== system Simulink_Vortex/Wheel Walking - Normal Driving/Wheel walking speed profile/Ideal turn radius/Half acceleration ==
  Constant : Constant
  Constant2 : Constant  Value=0.4
  Divide : Product  Inputs=*/
  Repeating Sequence : simulink/Sources/Repeating Sequence  rep_seq_t=[0.665 14.63 14.63+0.000001 15.96 15.96+0.000001]  rep_seq_y=[1 1 2 2 1]
  Subtract : Sum  Inputs=+-
  Acceleration : Outport
  wires:
  Constant/1 -> Subtract/2
  Subtract/1 -> Divide/1
  Repeating Sequence/1 -> Subtract/1
  Constant2/1 -> Divide/2
  Divide/1 -> Acceleration/1

== matlab function Simulink_Vortex/Real turn radius /1 ==
  data: xp input; yp input; v output
function v = globallinealspeed(xp,yp)
%#codegen
v = sqrt(yp^2+xp^2);

== matlab function Simulink_Vortex/Body Odometry/  ==
  data: r11 input; r12 input; r13 input; r21 input; r31 input; theta output; r32 input; r33 input; psi output; phi output
function [theta,psi,phi] = orientation(r11,r12,r13,r21,r31,r32,r33)

if (r31~= 1 && r31~=-1)
    theta= -asin(r31);
    psi = atan2(r32/cos(theta), r33/cos(theta));
    phi = atan2(r21/cos(theta), r11/cos(theta));
else
    phi = 0;
    if (r31 == -1)
        theta = pi/2;
        psi = phi + atan2(r12, r13);
    else
        theta = -pi/2;
        psi = -phi + atan2(-r12, -r13);
    end
end

== matlab function Simulink_Vortex/Body Odometry/1 ==
  data: xp input; yp input; v output; zp input
function v = globallinealspeed(xp,yp,zp)
%#codegen
v = sqrt(yp^2+xp^2+zp^2);

== matlab function Simulink_Vortex/Real turn radius /2 ==
  data: xp input; yp input; v output
function v = globallinealspeed(xp,yp)
%#codegen
v = sqrt(yp^2+xp^2);

== matlab function Simulink_Vortex/Wheel 2 Odometry1/  ==
  data: psi output; r11 input; r12 input; r13 input; r21 input; r22 input; theta output; r23 input; r33 input; phi output
function [psi,theta,phi] = orientation(r11,r12,r13,r21,r22,r23,r33)

ctheta = sqrt(r11^2+r12^2);
stheta = r13;
theta = atan2(stheta,ctheta);

if ctheta ~= 0
cphi = r11/ctheta;
sphi = -r12/ctheta;
phi = atan2(sphi,cphi);

cpsi = r33/ctheta;
spsi = -r23/ctheta;
psi = atan2(spsi,cpsi);
else
    if stheta >0
        cpp = r22;
        spp = r21;
        psi = 0;
        phi = atan2(spp,cpp);
    else
        cpp = r22;
        spp = r21;
        psi = 0;
        phi = atan2(spp,cpp);
    end
end

== matlab function Simulink_Vortex/Speed slip method/2 ==
  data: xp input; yp input; v output
function v = globallinealspeed(xp,yp)
%#codegen
v = sqrt(yp^2+xp^2);

== matlab function Simulink_Vortex/Wheel Walking - Normal Driving/Wheel walking speed profile/WW movement/MATLAB Function ==
  data: theta input; dx output; predx input
function dx = fcn(theta,predx)
dx = predx;
if predx > 0 && theta <15
    dx = predx;
elseif predx > 0 && theta >15
    dx = -predx;
elseif predx < 0 && theta >-15
    dx = predx;
elseif predx < 0 && theta <-15
    dx = -predx;
end

== matlab function Simulink_Vortex/Speed slip method/1 ==
  data: xp input; yp input; v output
function v = globallinealspeed(xp,yp)
%#codegen
v = sqrt(yp^2+xp^2);
